simulink model "PID_Controller"  (R2020a)
settings: Solver=ode15s  StartTime=0.0  StopTime=0.2  RelTol=1e-3
undefined symbols (not defined in the file): Kd, Ki, Kp
settings Model: DataDictionary=Motordata.sldd  Creator=NIKITA  LastModifiedBy=NIKITA
settings DataIOCC: SaveOutput=off  SaveTime=off

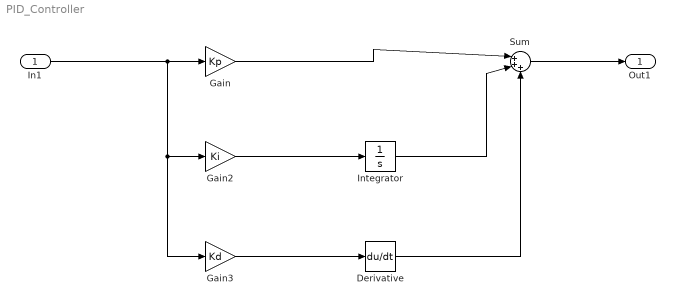
== system PID_Controller ==
  In1 : Inport  OutDataTypeStr=double  PortDimensions=1  SampleTime=[0,1]
  "Derivative " : Derivative
  Gain : Gain  Gain=Kp
  Gain2 : Gain  Gain=Ki
  Gain3 : Gain  Gain=Kd
  "Integrator " : Integrator
  Sum : Sum  Inputs=|+++
  Out1 : Outport  OutDataTypeStr=double  PortDimensions=1  SampleTime=0
  wires:
  Gain/1 -> Sum/1
  In1/1 -> Gain/1, Gain2/1, Gain3/1
  Sum/1 -> Out1/1
  Gain2/1 -> "Integrator "/1
  "Integrator "/1 -> Sum/2
  Gain3/1 -> "Derivative "/1
  "Derivative "/1 -> Sum/3
